simulink model "SimDisplay"  (R2024b)
settings: Solver=VariableStepAuto  StartTime=0.0  StopTime=10.0  RelTol=1e-3
undefined symbols (not defined in the file): Sim3dSensor
libraries: sim3dcameralib x1, sim3dlib x1, uavsim3dlib x1, sim3dgroundtruthsensorlib x1
settings Model: Creator=fears  LastModifiedBy=fears

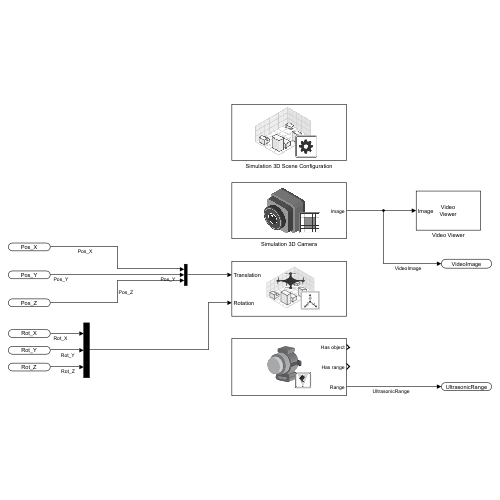
[thumbnail: Simulink's stored preview of the top-level diagram]
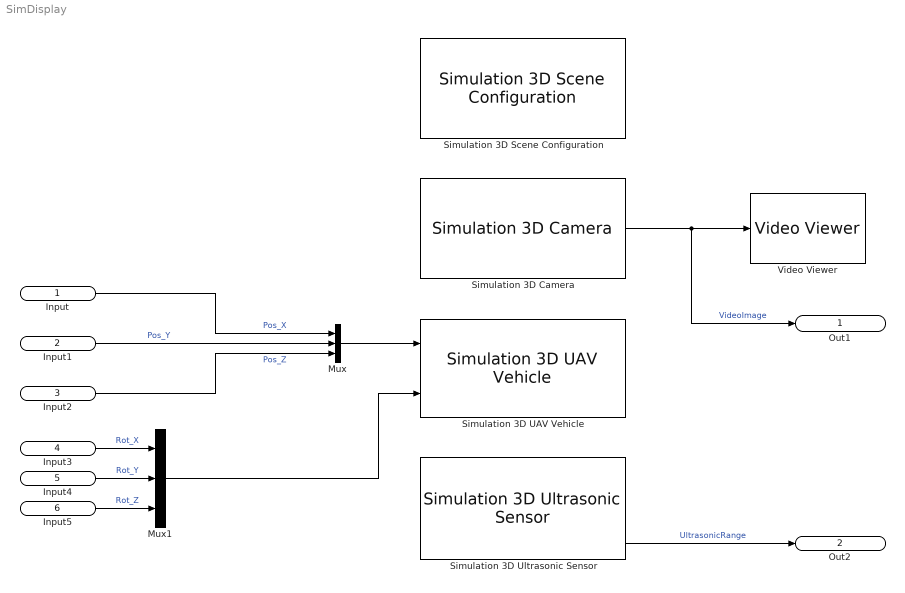
== system SimDisplay ==
  Input : Inport
  Input1 : Inport  Port=2
  Input2 : Inport  Port=3
  Input3 : Inport  Port=4
  Input4 : Inport  Port=5
  Input5 : Inport  Port=6
  Mux : Mux  Inputs=3
  Mux1 : Mux  Inputs=3
  Simulation 3D Camera : sim3dcameralib/Simulation 3D Camera  Priority=1  sensorTag=Sim3dSensor�  sensorId=1  sensorName=Sim3dSensor�  vehTagList={'Drone';'Scene Origin'}  vehTag=Drone  mountLoc=Origin  offsetFlag=on  tmountOffset=[0, 0, 0]  extTmount=off  rmountOffset=[0, 90, 0]  extRmount=off  FocalLength=[1109, 1109]  OpticalCenter=[640, 360]  ImageSize=[720, 1280]  RadialDistortion=[0, 0]  TangentialDistortion=[0, 0]  SensorSkew=0  DepthOutportEnabled=off  SemanticOutportEnabled=off  TransformOutportEnabled=off  SampleTime=-1  mountPoint=[0 0 0]  mountOrientation=[0 -90 0]  aMode=4  ID=1
      settings: LibrarySourceBlock=uavsim3dlib/Simulation 3D Camera
  Simulation 3D Scene Configuration : sim3dlib/Simulation 3D Scene Configuration  Priority=0  ProjectFormat=Unreal Editor  SceneDesc=US city block  ProjectName=D:\MATLAB\toolbox\shared\sim3d_projects\automotive_project_windows\UE\WindowsNoEditor\VehicleSimulation.exe  ScenePath=/Game/Maps/USCityBlock  UEProjPath=Unreal\AutoVrtlEnv\AutoVrtlEnv.uproject  EnableOpenDRIVE=off  vehTagList={'Custom';'Drone';'Scene Origin'}  vehTag=Custom  FreeCameraInitialTranslation=[0, 0, 0]  FreeCameraDefaultInitialTranslation=[-6, 0, 2]  FreeCameraInitialRotation=[0, 0, 0]  FreeCameraDefaultInitialRotation=[0, -15, 0]  OpVisEn=off  Ts=1/60  EnableWindow=on  EnableRemoteAccess=off  EnableWeather=off  SunAzimuth=90  SunAltitude=40.0  EnableGeospatialSun=off  Latitude=0  Longitude=0  Date=2023-01-01  Time=10:30:00  GeoTimeZone=-5.0  SunDaylightSaving=off  wind=1  clouds=10  EnableVolumetricClouds=off  CloudCoverage=0  CloudAltitude=6  fog=0  rain=0  RaindropsEffect=off  SnowDensity=0  EnableGeospatial=off  UseTrueOrigin=off  OriginHeight=200  OriginLatitude=40.744652  OriginLongitude=-73.988864  MapStyle=Aerial  AdditionalAssetIDs=[]  UseAdvancedSunSky=off  SolarTime=11  TimeZone=-5  Day=21  Month=9  Year=2022  UseDaylightSavingTime=on  DSTStartDay=10  DSTStartMonth=3  DSTEndDay=3  DSTEndMonth=11  DSTSwitchHour=2  sensorTag=MainCamera1  sensorId=1  sensorName=MainCamera1  mountLoc=Origin  offsetFlag=off  tmountOffset=[0, 0, 0]  rmountOffset=[0, 0, 0]  HorizontalResolution=1280  VerticalResolution=720  HorizontalFOV=60  mountPoint=[0 0 0]  mountOrientation=[0 0 0]  aMode=4  ID=1  GeoTrigger=Inactive
      settings: LibrarySourceBlock=uavsim3dlib/Simulation 3D Scene Configuration
  Simulation 3D UAV Vehicle : uavsim3dlib/Simulation 3D UAV Vehicle  Priority=-1  Mesh=Quadrotor  MeshPath=/MathWorksUAVContent/UAVs/HexaRotorUAV/HexaRotor.HexaRotor  Color=Black  ActorName=Drone  UseGlobalFrame=off  InitialTranslation=[0 0 0]  InitialRotation=[0 0 0]  InitialTranslationGlobal=[0 0 0]  InitialGeoOrigin=[0 0 0]  InitialRotationGlobal=[0 0 0]  SampleTime=-1  ActorType=SimulinkVehicle  ID=C  aMode=4  ActorTag=Drone
  Simulation 3D Ultrasonic Sensor : sim3dgroundtruthsensorlib/Simulation 3D Ultrasonic Sensor  Priority=1  sensorTag=Sim3dSensor�  sensorId=2  sensorName=Sim3dSensor�  vehTagList={'Drone';'Scene Origin'}  vehTag=Drone  mountLoc=Origin  offsetFlag=on  tmountOffset=[0, 0, 0]  rmountOffset=[0, 90, 0]  detectionRanges=[0.03 0.15 5.5]  HorizontalFoV=70  VerticalFoV=35  TransformOutportEnabled=off  SampleTime=-1  mountPoint=[0 0 0]  mountOrientation=[0 -90 0]  aMode=4  ID=2
      settings: LibrarySourceBlock=uavsim3dlib/Simulation 3D Ultrasonic Sensor
  Video Viewer : VideoViewer  FigPos=[229 786 418 304]
  Out1 : Outport
  Out2 : Outport  Port=2
  wires:
  Simulation 3D Camera/1 -> Out1/1, Video Viewer/1  "VideoImage"
  Mux/1 -> Simulation 3D UAV Vehicle/1
  Input/1 -> Mux/1  "Pos_X"
  Input2/1 -> Mux/3  "Pos_Z"
  Mux1/1 -> Simulation 3D UAV Vehicle/2
  Input1/1 -> Mux/2  "Pos_Y"
  Input3/1 -> Mux1/1  "Rot_X"
  Input4/1 -> Mux1/2  "Rot_Y"
  Input5/1 -> Mux1/3  "Rot_Z"
  Simulation 3D Ultrasonic Sensor/3 -> Out2/1  "UltrasonicRange"
